simulink library "powerlib"  (Simulink 6.0)
settings: Solver=ode45  SolverMode=SingleTasking  StartTime=0.0  StopTime=10.0  RelTol=1e-3
undefined symbols (not defined in the file or in its folder): com, ctrl1, Da, DiscIntNeverNeededParam, dtha, etat, FA, find_system, Ha, j, Ka, Ki, Kv, q0, Rground, sel, st_a, st_b, st_c, sta, stb, stc, T1, T2, T3, T4
libraries: powerlib_models x30, powerlib x25, simulink_extras x6, powerlib_extras x3, simulink x2
(part 1 of 7)
Description:
  | SimPowerSystems 3.1 block library.
  | 
  | Copyright  1997-2004 TransEnergie Technologies,
  | 
  | under sublicense from Hydro-Quebec,
  | 
  | and The MathWorks, Inc.
settings Model: Creator=Patrice Brunelle  ModifiedByFormat=Patrice Brunelle  LastModifiedBy=Patrice Brunelle  ExtModeAutoUpdateStatusClock=off
settings Model: ModifiedHistory=|
  | Latest modifications :
  | 
  | - Fix the DC Machine Discrete block:
  |   change the SampleTime parameter to: Ts
  | - Update the preset model parameters list.
settings DataIOCC: SignalLoggingName=logsOut
settings OptimizationCC: BooleanDataType=off
settings DebuggingCC: CheckExecutionContextPreStartOutputMsg=on  CheckExecutionContextRuntimeOutputMsg=on  SolverPrmCheckMsg=none
settings HardwareCC: TargetUnknown=on
settings ModelReferenceCC: UpdateModelReferenceTargets=IfOutOfDate

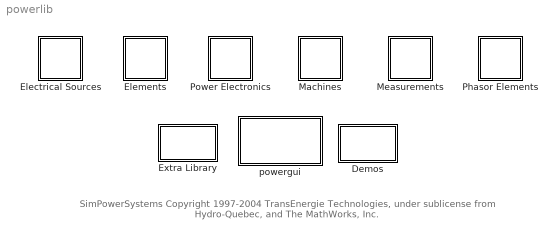
== system powerlib ==
  note: SimPowerSystems
      | Copyright  1997-2004 TransEnergie Technologies, under sublicense
      | from Hydro-Quebec, and The MathWorks, Inc.
  Demos : Subsystem
      settings: OpenFcn=demo('Simulink','SimPowerSystems')
      mask Display: disp('Demos')
  Electrical Sources : Subsystem  Opaque=on
      mask init:
      | powerlibroot = which('powersysdomain');
      | PSBroot = powerlibroot(1:end-16);
      mask Display: image(imread([PSBroot,'PSBsources.bmp'],'bmp'))
  Elements : Subsystem
      mask init:
      | powerlibroot = which('powersysdomain');
      | PSBroot = powerlibroot(1:end-16);
      mask Display: image(imread([PSBroot,'PSBelements.bmp'],'bmp'))
  Extra Library : Subsystem
      settings: OpenFcn=powerlib_extras
      mask Display: disp('Extras')
  Machines : Subsystem
      mask init:
      | powerlibroot = which('powersysdomain');
      | PSBroot = powerlibroot(1:end-16);
      mask Display: image(imread([PSBroot,'PSBmachines.bmp'],'bmp'))
  Measurements : Subsystem
      mask init:
      | powerlibroot = which('powersysdomain');
      | PSBroot = powerlibroot(1:end-16);
      mask Display: image(imread([PSBroot,'PSBmeasurements.bmp'],'bmp'))
  Phasor Elements : Subsystem
      mask init:
      | powerlibroot = which('powersysdomain');
      | PSBroot = powerlibroot(1:end-16);
      mask Display: image(imread([PSBroot,'PSBphasors.bmp'],'bmp'))
  Power Electronics : Subsystem
      mask init:
      | powerlibroot = which('powersysdomain');
      | PSBroot = powerlibroot(1:end-16);
      mask Display: image(imread([PSBroot,'PSBelectronics.bmp'],'bmp'))
  powergui : Subsystem  Priority=2  mask(PSB option menu block){Frange=[0:2:500], Ylog=off, Xlog=on, save=off, variable=ZData, structure=, ZoomFFT=on, StartTime=0.0, cycles=1, DisplayStyle=1, fundamental=60, FreqAxis=off, MaxFrequency=1000, frequencyindice=1, frequencyindicesteady=1, RmsSteady=1, display=off, Ts=0, methode=off, frequency=60, echomessages=off}
      mask prompts: Frange "Frequency Range (PSBZMETER)"; Ylog "Log impedance (PSBZMETER)"; Xlog "log Frequency (PSBZMETER)"; save "Save Data To Workspace (PSBZMETER)"; variable "Variable Name (PSBZMETER)"; structure "Structure Name (PSBFFTSCOPE)"; ZoomFFT "ZoomFFT (PSBFFTSCOPE)"; StartTime "Start Time (PSBFFTSCOPE)"; cycles "Cycles (PSBFFTSCOPE)"; DisplayStyle "Display style (PSBFFTSCOPE)"; fundamental "Fundamental (PSBFFTSCOPE)"; FreqAxis "Frequency Axis (PSBFFTSCOPE)"; MaxFrequency "Max Frequency (PSBFFTSCOPE)"; frequencyindice "Frequency indice  (PSBLOADFLOW)"; frequencyindicesteady "Frequency indice (STEADYSTATE)"; RmsSteady "RMS display (STEADYSTATE)"; display "Display Results"; Ts "Sample time (s):"; methode "Phasor simulation"; frequency "phasor frequency"; echomessages "Echo initialisation messages"
      mask init:
      | powerlibroot = which('powersysdomain');
      | PSBroot = powerlibroot(1:end-16);
      | if isempty(Ts);Ts=-1;end;
      | if Ts==0
      |   message=sprintf('Continuous');
      | elseif Ts>0
      |   message=sprintf('Discrete,\nTs = %.4g s.',Ts);
      | else
      |   message=sprintf('Discrete,\n Ts = ?');
      | end
      | if methode
      |     message=sprintf('Phasors');
      | end
      | if strcmp(bdroot,'powerlib')
      |   message='powergui';
      | end
      settings: CopyFcn=powergui('Copy_Callback',gcb,0,[]);  DeleteFcn=powergui('Copy_Callback',gcb,1,[]);powergui('Close_Callback',gcb,[],[]);  ModelCloseFcn=powergui('Close_Callback',gcb,[],[]);  OpenFcn=powergui(gcb,'PM')
      settings: PreSaveFcn=|
      | try
      | close(get_param(gcbh,'userdata'))
      | end
      mask Help: web(psbhelp)
      mask Display:
      | image(imread([PSBroot,'PSBpowergui.bmp'],'bmp'))
      | disp(message)

== system powerlib/Demos ==

== system powerlib/Electrical Sources ==
  AC Current Source : Subsystem  Orientation=up  mask(AC Current Source){Amplitude=10, Phase=0, Frequency=60, SampleTime=0, Measurements=None}
      mask prompts: Amplitude "Peak amplitude (A):"; Phase "Phase (deg):"; Frequency "Frequency (Hz):"; SampleTime "Sample time:"
      mask help: Ideal sinusoidal AC current source. The positive current direction is indicated by the arrow.
      mask init:
      | block = gcb;
      | powericon('psbloadfunction',block,'goto','Initialize');
      | powericon('ACSourceInit',block);
      settings: CopyFcn=powericon('psbloadfunction',gcb,'goto','UpdateGotoTag');
      mask Help: web(psbhelp);
      mask StyleString: edit,edit,edit,edit,popup(None|Current)
      mask Display: plot(-50,-35,50,50-15,[0,9,18,24,29,30,29,24,18,9,0,-9,-18,-24,-29,-30,-29,-24,-18,-9,0],[30,29,24,18,9,0,-9,-18,-24,-29,-30,-29,-24,-18,-9,0,9,18,24,29,30],[-20 5 5 20 5 5],[2 2 12 2 -8 2],[-50 -30],[0 0],[50,30],[0 0],[45 35 40 40 40],[15 15 15 20 10]);
  AC Voltage Source : Subsystem  Orientation=up  mask(AC Voltage Source){Amplitude=100, Phase=0, Frequency=60, SampleTime=0, Measurements=None}
      mask prompts: Amplitude "Peak amplitude (V):"; Phase "Phase (deg):"; Frequency "Frequency (Hz):"; SampleTime "Sample time:"
      mask help: Ideal sinusoidal AC Voltage source.
      mask init:
      | block=gcb;
      | powericon('psbloadfunction',block,'goto','Initialize');
      | powericon('ACSourceInit',block);
      settings: CopyFcn=powericon('psbloadfunction',gcb,'goto','UpdateGotoTag');
      mask Help: web(psbhelp);
      mask StyleString: edit,edit,edit,edit,popup(None|Voltage)
      mask Display: plot(-50,-35,50,50-15,[0,9,18,24,29,30,29,24,18,9,0,-9,-18,-24,-29,-30,-29,-24,-18,-9,0],[30,29,24,18,9,0,-9,-18,-24,-29,-30,-29,-24,-18,-9,0,9,18,24,29,30],[-50 -30],[0 0],[50,30],[0 0],[45 35 40 40 40],[15 15 15 20 10],[0,9,18,24,29,30,29,24,18,9,0,-9,-18,-24,-29,-30,-29,-24,-18,-9,0]./-2.4,[1 2 3 4 5 6 7 8 9 10 11 12 13 14 15 16 17 18 19 20 21].*1.5-15);
  Controlled Current Source : Subsystem  Orientation=up  mask(Controlled Current Source){Initialize=on, SourceType=AC, Amplitude=0, Phase=0, Frequency=0, Measurements=None}
      mask prompts: SourceType "Source type"; Amplitude "Initial amplitude (A):"; Phase "Initial phase (deg):"; Frequency "Initial frequency (Hz):"
      mask help:
      | Converts the Simulink input signal into an equivalent current source. The generated current is driven by the input signal of the block.
      |
      | You can initialize your circuit with a specific AC or DC current. If you want to start the simulation in steady-state, the block input must be connected to a signal starting as a sinusoidal or DC waveform corresponding to the initial values.
      mask init:
      | powericon('psbloadfunction',gcb,'goto','Initialize');
      settings: CopyFcn=powericon('psbloadfunction',gcb,'goto','UpdateGotoTag');
      mask Help: web(psbhelp);
      mask StyleString: checkbox,popup(AC|DC),edit,edit,edit,popup(None|Current)
      mask CallbackString: powericon('ControlledSourcesCback',gcb);|powericon('ControlledSourcesCback',gcb);||||
      mask Display: plot(-50,-35,50,50-15,[0,9,18,24,29,30,29,24,18,9,0,-9,-18,-24,-29,-30,-29,-24,-18,-9,0],[30,29,24,18,9,0,-9,-18,-24,-29,-30,-29,-24,-18,-9,0,9,18,24,29,30],[-20 5 5 20 5 5],[2 2 12 2 -8 2]);
  Controlled Voltage Source : Subsystem  Orientation=up  mask(Controlled Voltage Source){Initialize=on, SourceType=AC, Amplitude=0, Phase=0, Frequency=0, Measurements=None}
      mask prompts: SourceType "Source type"; Amplitude "Initial amplitude (V):"; Phase "Initial phase (deg):"; Frequency "Initial frequency (Hz):"
      mask help:
      | Converts the Simulink input signal into an equivalent voltage source. The generated voltage is driven by the input signal of the block.
      |
      | You can initialize your circuit with a specific AC or DC voltage. If you want to start the simulation in steady-state, the block input must be connected to a signal starting as a sinusoidal or DC waveform corresponding to the initial values.
      mask init:
      | powericon('psbloadfunction',gcb,'goto','Initialize');
      settings: CopyFcn=powericon('psbloadfunction',gcb,'goto','UpdateGotoTag');
      mask Help: web(psbhelp);
      mask StyleString: checkbox,popup(AC|DC),edit,edit,edit,popup(None|Voltage)
      mask CallbackString: powericon('ControlledSourcesCback',gcb);|powericon('ControlledSourcesCback',gcb);||||
      mask Display: plot(-50,-35,50,50-15,[0,9,18,24,29,30,29,24,18,9,0,-9,-18,-24,-29,-30,-29,-24,-18,-9,0],[30,29,24,18,9,0,-9,-18,-24,-29,-30,-29,-24,-18,-9,0,9,18,24,29,30],[0,9,18,24,29,30,29,24,18,9,0,-9,-18,-24,-29,-30,-29,-24,-18,-9,0]./-2.4,[1 2 3 4 5 6 7 8 9 10 11 12 13 14 15 16 17 18 19 20 21].*1.5-15);
  DC Voltage Source : Subsystem  Orientation=up  mask(DC Voltage Source){Amplitude=100, Measurements=None}
      mask prompts: Amplitude "Amplitude (V):"
      mask help: Ideal DC voltage source.
      mask init:
      | block=gcb;
      | powericon('psbloadfunction',block,'goto','Initialize');
      | powericon('DCVoltageSourceInit',block);
      settings: CopyFcn=powericon('psbloadfunction',gcb,'goto','UpdateGotoTag');
      mask Help: web(psbhelp);
      mask StyleString: edit,popup(None|Voltage)
      mask Display: plot(-10,-5,10,5,[10 1.25 1.25 1.25],[0 0 5 -5],[-10 -1.25 -1.25 -1.25],[0 0 -2 2],[6 4 5 5 5],[3 3 3 4 2])
  Three-Phase Programmable Voltage Source : Subsystem  mask(Three-Phase Programmable Voltage Source){PositiveSequence=[100  0 60], VariationEntity=Amplitude, VariationType=Step, VariationStep=0.5, VariationRate=10, VariationMagnitude=0.3, VariationFrequency=2, VariationTiming=[1 2], VariationPhaseA=off, Amplitudes=[1 0.8 1.2 1.0], TimeValues=[0 0.1 0.15 0.2], HarmonicGeneration=off, HarmonicA=[3 0.2 -25 0], HarmonicB=[2 0.15 35 2], Timing=[0.05  3]}
      mask prompts: PositiveSequence "Positive-sequence: [ Amplitude(Vrms Ph-Ph)  Phase(deg.)   Freq. (Hz) ]"; VariationEntity "Time variation of:"; VariationType "Type of variation:"; VariationStep "Step magnitude (pu, Hz or deg.):"; VariationRate "Rate of change (pu/s, Hz/s or deg/s):"; VariationMagnitude "Amplitude of the modulation (pu, Hz or deg.):"; VariationFrequency "Frequency of the modulation(Hz):"; VariationTiming "Variation timing (s) : [ Start   End ]"; VariationPhaseA "Variation on phase A only"; Amplitudes "Amplitude values (pu):"; TimeValues "Time values:"; HarmonicGeneration "Fundamental and/or Harmonic generation:"; HarmonicA "A:  [ Order(n)   Amplitude(pu) Phase(degrees)  Seq(0, 1 or 2) ]"; HarmonicB "B:  [ Order(n)   Amplitude(pu) Phase(degrees)  Seq(0, 1 or 2) ]"; Timing "Timing (s) : [ Start   End ]"
      mask help:
      | This block implements a three-phase zero-impedance voltage source. The common node (neutral) of the three sources is accessible via input 1 (N) of the block. Time variation for the amplitude, phase and frequency of the fundamental can be pre-programmed. In addition, two harmonics can be surimposed on the fundamental.
      |
      | Note: For  "Phasor simulation" , frequency variation and harmonic injection are not allowed.  Specify  Order =1 and Seq=1,2 or 0 to inject additional fundamendal components A and B in  any sequence.
      mask init:
      | block=gcb;
      | % Extra variable:
      | SinglePhase=0;
      | 
      | % Conversion of pos. seq.amplitude from Ph-Ph rms voltage to Phase-gnd peak
      | MagnitudeVps = PositiveSequence(1)*sqrt(2/3);
      | PhaseVps = PositiveSequence(2);
      | FreqVps = PositiveSequence(3);
      | 
      | % Conversion of harmonic amplitudes from pu to Phase-gnd peak volt
      | HarmonicA(2) = HarmonicA(2)*MagnitudeVps;
      | HarmonicB(2) = HarmonicB(2)*MagnitudeVps;
      | 
      | % Conversion of amplitude variation from pu to Ph-G peak volt
      | if VariationEntity==2
      | 	VariationStep = VariationStep*MagnitudeVps;
      | 	VariationRate = VariationRate*MagnitudeVps;
      | 	VariationMagnitude  = VariationMagnitude*MagnitudeVps;
      | 	Amplitudes = Amplitudes*MagnitudeVps;
      | end
      | 
      | % extract other parameters
      | Ton_Variation = VariationTiming(1);
      | Toff_Variation = VariationTiming(2);
      | %
      | n_HarmoA = HarmonicA(1);
      | Mag_HarmoA = HarmonicA(2);
      | Phase_HarmoA = HarmonicA(3);
      | Seq_HarmoA = HarmonicA(4);
      | if n_HarmoA==0
      |     Phase_HarmoA = 90;
      |     Seq_HarmoA = 0;
      | end
      | %
      | n_HarmoB = HarmonicB(1);
      | Mag_HarmoB = HarmonicB(2);
      | Phase_HarmoB = HarmonicB(3);
      | Seq_HarmoB = HarmonicB(4);
      | if n_HarmoB==0
      |     Phase_HarmoB = 90;
      |     Seq_HarmoB = 0;
      | end
      | %
      | Ton_Harmo = Timing(1);
      | Toff_Harmo = Timing(2);
      | %
      | if TimeValues(1)~=0,
      |     TimeValues=[0 TimeValues];
      |     Amplitudes=[0 Amplitudes];
      | end
      | %
      | n = length(TimeValues); 
      | vec_dt = [TimeValues,0] - [0,TimeValues];
      | vec_dt = vec_dt(2:n);
      | %
      | powericon('psbloadfunction',block,'goto','Initialize');
      | Ts = powericon('ThreePhaseProgSourceInit',block);
      settings: CopyFcn=powericon('psbloadfunction',gcb,'goto','UpdateGotoTag');
      mask Help: web(psbhelp)
      mask StyleString: edit,popup(None|Amplitude|Phase|Frequency),popup(Step|Ramp|Modulation|Table of time-amplitude pairs),edit,edit,edit,edit,edit,checkbox,edit,edit,checkbox,edit,edit,edit
      mask CallbackString: |powericon('ProgrammableVoltageSourceCback',gcb);|powericon('ProgrammableVoltageSourceCback',gcb);|||||||||powericon('ProgrammableVoltageSourceCback',gcb);|||
      mask Display: plot(-80,-50,80,50,[0,9,18,24,29,30,29,24,18,9,0,-9,-18,-24,-29,-30,-29,-24,-18,-9,0],[30,29,24,18,9,0,-9,-18,-24,-29,-30,-29,-24,-18,-9,0,9,18,24,29,30],[-50 -30],[0 0],[50,30],[0 0],[45 35 40 40 40],[15 15 15 20 10],[1 2 3 4 5 6 7 8 9 10 11 12 13 14 15 16 17 18 19 20 21].*1.5-15,[0,9,18,24,29,30,29,24,18,9,0,-9,-18,-24,-29,-30,-29,-24,-18,-9,0]./2.4)
  Three-Phase Source : Subsystem  mask(Three-Phase Source){Voltage=25e3, PhaseAngle=0, Frequency=60, InternalConnection=Yg, SpecifyImpedance=on, Resistance=0.8929, Inductance=16.58e-3, ShortCircuitLevel=100e6, BaseVoltage=25e3, XRratio=7}
      mask prompts: Voltage "Phase-to-phase rms voltage (V):"; PhaseAngle "Phase angle of phase A (degrees):"; Frequency "Frequency (Hz):"; InternalConnection "Internal connection:"; SpecifyImpedance "Specify impedance using short-circuit level"; Resistance "Source resistance (Ohms):"; Inductance "Source inductance (H):"; ShortCircuitLevel "3-phase short-circuit level at base voltage(VA):"; BaseVoltage "Base voltage (Vrms ph-ph):"; XRratio "X/R ratio:"
      mask help: Three-phase voltage source in series with RL branch.
      mask init:
      | block = gcb;
      | Amplitude = Voltage*sqrt(2)/sqrt(3);
      | Phase=PhaseAngle;
      | powericon('ThreePhaseSourceCback',block);
      | [s1,s2,s3,s4,g1,g2,g3,g4,g5,g6] = powericon('ThreePhaseSourceIcon',Resistance,Inductance,InternalConnection);
      | powericon('psbloadfunction',block,'goto','Initialize');
      | Ts = powericon('ThreePhaseSourceInit',block);
      settings: CopyFcn=powericon('psbloadfunction',gcb,'goto','UpdateGotoTag');
      mask Help: web(psbhelp);
      mask StyleString: edit,edit,edit,popup(Y|Yn|Yg),checkbox,edit,edit,edit,edit,edit
      mask CallbackString: |||powericon('ThreePhaseSourceCback',gcb);|powericon('ThreePhaseSourceCback',gcb);|||||
      mask Display:
      | plot(-180,-50,350,50,s1,s2,s3,s4,
      | [0,9,18,24,29,30,29,24,18,9,0,-9,-18,-24,-29,-30,-29,-24,-18,-9,0]*1.5-45,
      | [30,29,24,18,9,0,-9,-18,-24,-29,-30,-29,-24,-18,-9,0,9,18,24,29,30]*0.8,[-150,-90],[0,0]);
      | plot(g1,g2,g3,g4,g5,g6);
      | plot([1 2 3 4 5 6 7 8 9 10 11 12 13 14 15 16 17 18 19 20 21].*2.5-72,
      | [0,9,18,24,29,30,29,24,18,9,0,-9,-18,-24,-29,-30,-29,-24,-18,-9,0]./3)
